simulink model "EHA_Sine"  (R2018a)
settings: Solver=VariableStepAuto  StartTime=0.0  StopTime=2  RelTol=1e-3
undefined symbols (not defined in the file): A, b, beta, Kv, L, m, P_r, P_s, V0, wn, zeta
settings Model: Creator=UFUK  LastModifiedBy=UFUK

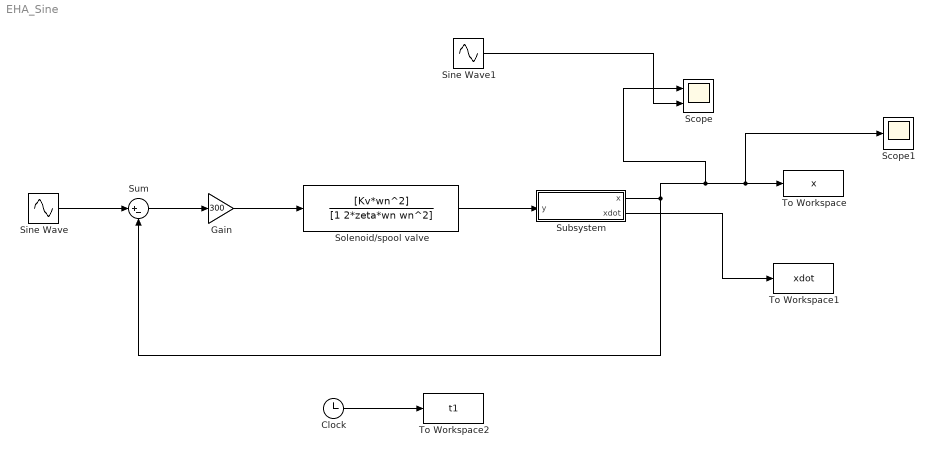
== system EHA_Sine ==
  Clock : Clock
  Gain : Gain  Gain=300
  Scope : Scope  NumInputPorts=2
  Scope1 : Scope
  Sine Wave : Sin  Amplitude=L/4  Bias=L/2  Frequency=12.56  SampleTime=0
  Sine Wave1 : Sin  Amplitude=0.17  Bias=0.34  Frequency=12.56  SampleTime=0
  Solenoid/spool valve : TransferFcn  Numerator=[Kv*wn^2]  Denominator=[1 2*zeta*wn wn^2]
  Subsystem : Subsystem
  Sum : Sum  Inputs=|+-
  To Workspace : ToWorkspace  VariableName=x  SaveFormat=Timeseries  SampleTime=-1
  To Workspace1 : ToWorkspace  VariableName=xdot  SaveFormat=Timeseries  SampleTime=-1
  To Workspace2 : ToWorkspace  VariableName=t1  SaveFormat=Timeseries  SampleTime=-1
  wires:
  Gain/1 -> Solenoid/spool valve/1
  Solenoid/spool valve/1 -> Subsystem/1("y ")
  Sum/1 -> Gain/1
  Clock/1 -> To Workspace2/1
  Subsystem/2(xdot) -> To Workspace1/1
  Sine Wave/1 -> Sum/1
  Subsystem/1(x) -> Scope/1, Scope1/1, To Workspace/1, Sum/2
  Sine Wave1/1 -> Scope/2

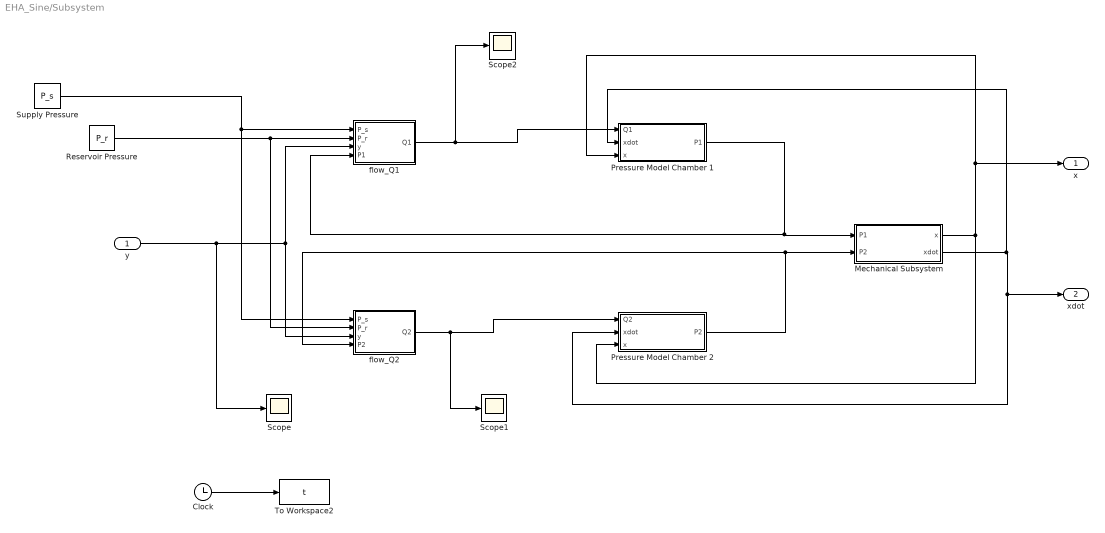
== system EHA_Sine/Subsystem ==
  "y " : Inport
  Clock : Clock
  "Mechanical Subsystem " : Subsystem
  Pressure Model Chamber 1 : Subsystem
  "Pressure Model Chamber 2 " : Subsystem
  Reservoir Pressure : Constant  Value=P_r
  Scope : Scope
  Scope1 : Scope
  Scope2 : Scope
  Supply Pressure : Constant  Value=P_s
  To Workspace2 : ToWorkspace  VariableName=t  SaveFormat=Timeseries  SampleTime=-1
  "flow_Q1 " : MATLAB Function  TreatAsAtomicUnit=on
  "flow_Q2 " : MATLAB Function  TreatAsAtomicUnit=on
  x : Outport
  xdot : Outport  Port=2
  wires:
  "y "/1 -> Scope/1, "flow_Q2 "/3(y), "flow_Q1 "/3(y)
  Supply Pressure/1 -> "flow_Q2 "/1(P_s), "flow_Q1 "/1(P_s)
  Reservoir Pressure/1 -> "flow_Q2 "/2(P_r), "flow_Q1 "/2(P_r)
  Pressure Model Chamber 1/1(P1) -> "flow_Q1 "/4(P1), "Mechanical Subsystem "/1(P1)
  "Pressure Model Chamber 2 "/1(P2) -> "flow_Q2 "/4(P2), "Mechanical Subsystem "/2(P2)
  "Mechanical Subsystem "/1(x) -> "Pressure Model Chamber 2 "/3(x), x/1, Pressure Model Chamber 1/3(x)
  "Mechanical Subsystem "/2(xdot) -> Pressure Model Chamber 1/2(xdot), xdot/1, "Pressure Model Chamber 2 "/2(xdot)
  "flow_Q2 "/1(Q2) -> Scope1/1, "Pressure Model Chamber 2 "/1(Q2)
  "flow_Q1 "/1(Q1) -> Scope2/1, Pressure Model Chamber 1/1(Q1)
  Clock/1 -> To Workspace2/1

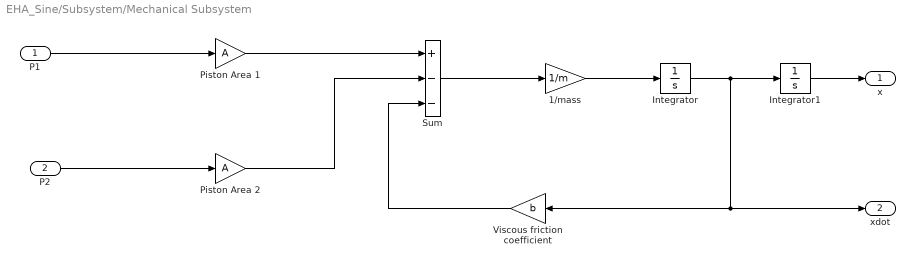
== system EHA_Sine/Subsystem/Mechanical Subsystem  ==
  P1 : Inport
  P2 : Inport  Port=2
  1/mass : Gain  Gain=1/m
  Integrator : Integrator
  Integrator1 : Integrator  InitialCondition=L/2
  Piston Area 1 : Gain  Gain=A
  Piston Area 2 : Gain  Gain=A
  Sum : Sum  Inputs=+--  OutMin=[1]  OutMax=[3]
  Viscous friction coefficient : Gain  Gain=b
  x : Outport
  xdot : Outport  Port=2
  wires:
  Piston Area 2/1 -> Sum/2
  Piston Area 1/1 -> Sum/1
  1/mass/1 -> Integrator/1
  Integrator1/1 -> x/1
  Viscous friction coefficient/1 -> Sum/3
  P2/1 -> Piston Area 2/1
  P1/1 -> Piston Area 1/1
  Sum/1 -> 1/mass/1
  Integrator/1 -> Viscous friction coefficient/1, xdot/1, Integrator1/1

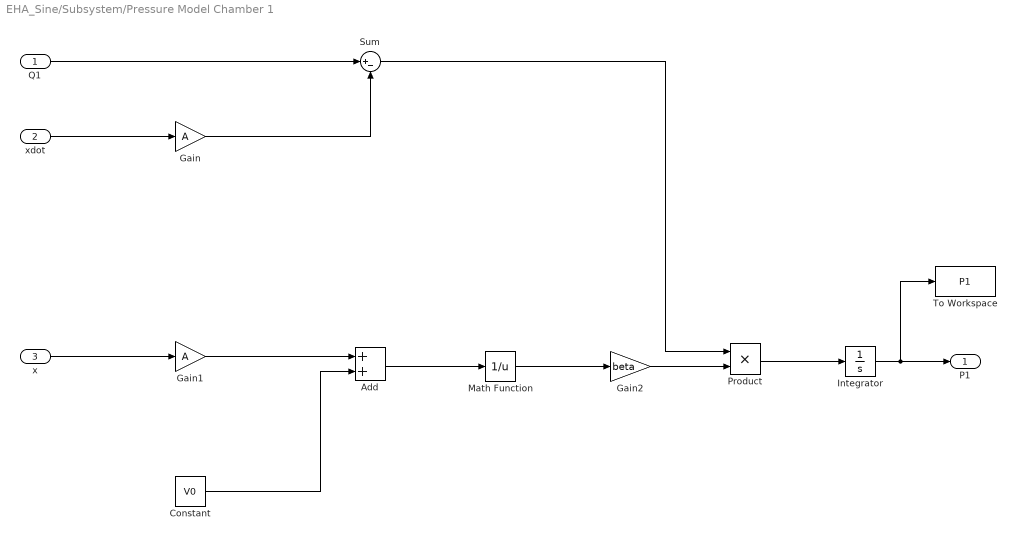
== system EHA_Sine/Subsystem/Pressure Model Chamber 1 ==
  Q1 : Inport
  xdot : Inport  Port=2
  x : Inport  Port=3
  Add : Sum
  Constant : Constant  Value=V0
  Gain : Gain  Gain=A
  Gain1 : Gain  Gain=A
  Gain2 : Gain  Gain=beta
  Integrator : Integrator  InitialCondition=0.1*P_s
  Math Function : Math  Operator=reciprocal  SaturateOnIntegerOverflow=on
  Product : Product
  Sum : Sum  Inputs=|+-
  To Workspace : ToWorkspace  VariableName=P1  SaveFormat=Timeseries  SampleTime=-1
  P1 : Outport
  wires:
  Q1/1 -> Sum/1
  xdot/1 -> Gain/1
  Gain/1 -> Sum/2
  x/1 -> Gain1/1
  Constant/1 -> Add/2
  Gain1/1 -> Add/1
  Add/1 -> Math Function/1
  Math Function/1 -> Gain2/1
  Gain2/1 -> Product/2
  Sum/1 -> Product/1
  Integrator/1 -> To Workspace/1, P1/1
  Product/1 -> Integrator/1

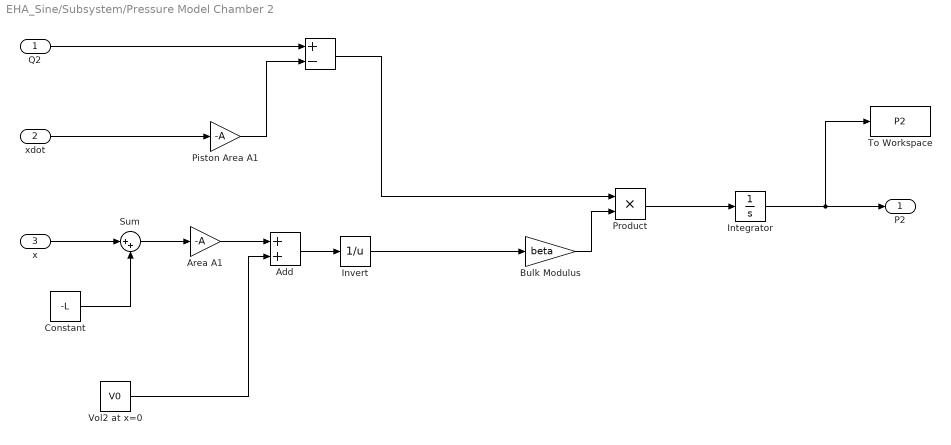
== system EHA_Sine/Subsystem/Pressure Model Chamber 2  ==
  Q2 : Inport
  xdot : Inport  Port=2
  x : Inport  Port=3
  " " : Sum  Inputs=+-
  Add : Sum
  Area A1 : Gain  Gain=-A
  Bulk Modulus : Gain  Gain=beta
  Constant : Constant  Value=-L
  Integrator : Integrator  InitialCondition=0.1*P_s
  Invert : Math  Operator=reciprocal  SaturateOnIntegerOverflow=on
  Piston Area A1 : Gain  Gain=-A
  Product : Product
  Sum : Sum  Inputs=|++
  To Workspace : ToWorkspace  VariableName=P2  SaveFormat=Timeseries  SampleTime=-1
  Vol2 at x=0 : Constant  Value=V0
  P2 : Outport
  wires:
  Integrator/1 -> P2/1, To Workspace/1
  " "/1 -> Product/1
  Bulk Modulus/1 -> Product/2
  Add/1 -> Invert/1
  Area A1/1 -> Add/1
  Vol2 at x=0/1 -> Add/2
  Piston Area A1/1 -> " "/2
  Q2/1 -> " "/1
  x/1 -> Sum/1
  xdot/1 -> Piston Area A1/1
  Invert/1 -> Bulk Modulus/1
  Product/1 -> Integrator/1
  Constant/1 -> Sum/2
  Sum/1 -> Area A1/1

== matlab function EHA_Sine/Subsystem/flow_Q2  ==
  data: P_s input; Q2 output; P_r input; y input; P2 input
function Q2 = flow_Q2(P_s,P_r,y,P2)
u = [P_s,P_r,y,P2];
% system parameter
h = 0.009; % height of valve opening, m
% hydraulic constants
Cd = 0.68; % discharge coefficient
rho = 893; % fluid density, kg/m^3
% System inputs
P_s = u(1); % supply pressure, Pa
P_r = u(2); % reservoir pressure, Pa
y = u(3); % valve displacement, m
P2 = u(4); % pressure in chamber 2, Pa
% Compute valve orifice area
Av = abs(y)*h; % valve orifice area, m^2
if y <= 0
Q2 =Cd*Av*sign(P_s-P2)*sqrt( 2*abs(P_s-P2)/rho );
else
Q2 =-Cd*Av*sign(P2-P_r)*sqrt( 2*abs(P2-P_r)/rho );
end
y=u;

== matlab function EHA_Sine/Subsystem/flow_Q1  ==
  data: P_s input; Q1 output; P_r input; y input; P1 input
function Q1 = flow_Q1(P_s,P_r,y,P1)
u = [P_s,P_r,y,P1]';
% system parameter
h = 0.009; % height of valve opening, m
% hydraulic constants
Cd = 0.68; % discharge coefficient
rho = 893; % fluid density, kg/m^3
% System inputs
P_s = u(1); % supply pressure, Pa
P_r = u(2); % reservoir pressure, Pa
y = u(3); % valve displacement, m
P1 = u(4); % pressure in chamber 1, Pa
% Compute valve orifice area
Av = abs(y)*h; % valve orifice area, m^2
if y >= 0
Q1 = Cd*Av*sign(P_s-P1)*sqrt(2*abs(P_s-P1)/rho);
else
Q1 = -Cd*Av*sign(P1-P_r)*sqrt(2*abs(P1-P_r)/rho);
end
y=u;
